simulink model "Different_Functions"  (R2025b)
settings: Solver=FixedStepDiscrete  StartTime=0.0  StopTime=10.0  FixedStep=0.01  RelTol=1e-3
libraries: simulink x1
settings Model: Creator=soura  LastModifiedBy=soura

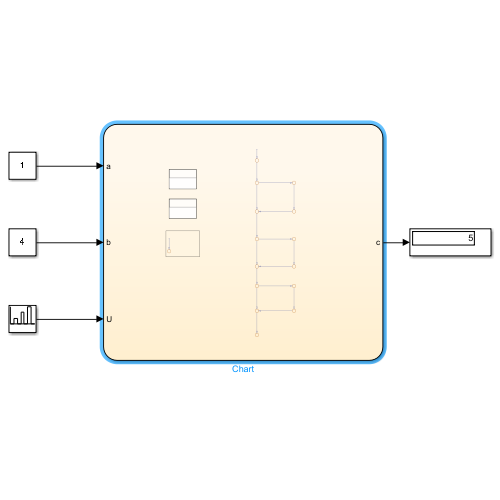
[thumbnail: Simulink's stored preview of the top-level diagram]
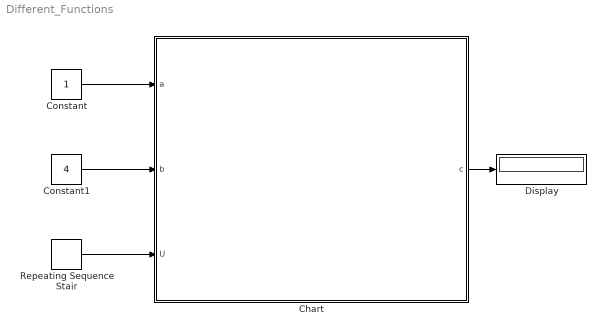
== system Different_Functions ==
  Chart : Stateflow chart  TreatAsAtomicUnit=on
  Constant : Constant  OutDataTypeStr=uint8
  Constant1 : Constant  Value=4  OutDataTypeStr=uint8
  Display : Display
  Repeating Sequence Stair : simulink/Sources/Repeating Sequence Stair  OutValues=[0 1 0 2 0 3 0].'  tsamp=-1  OutMin=[]  OutMax=[]  OutDataTypeStr=double  OutputDataTypeScalingMode=double  OutDataType=fixdt(0,8)  ConRadixGroup=Best Precision: Vector-wise  OutScaling=2^-12
  wires:
  Constant/1 -> Chart/1(a)
  Constant1/1 -> Chart/2(b)
  Repeating Sequence Stair/1 -> Chart/3(U)
  Chart/1(c) -> Display/1

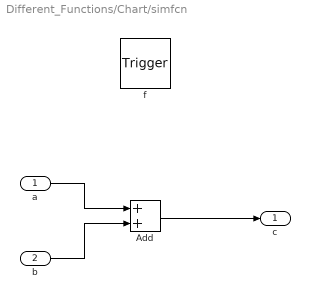
== system Different_Functions/Chart/simfcn ==
  a : Inport  OutDataTypeStr=uint8  PortDimensions=1
  b : Inport  Port=2  OutDataTypeStr=uint8  PortDimensions=1
  f : TriggerPort  TriggerType=function-call  VariantControl=(inherit)
      settings: CopyFcn=Stateflow.SLINSF.SimulinkMan.removeBlockPreDeleteFcn  PreDeleteFcn=Stateflow.SLINSF.SimulinkMan.unsafePredeleteFcn
  Add : Sum
  c : Outport
  wires:
  a/1 -> Add/1
  b/1 -> Add/2
  Add/1 -> c/1

== stateflow chart Different_Functions/Chart ==
  state c = simfcn(a,b) [function]
  state c=add1(a,b) [function]
    (default) -> (junction 14) : {c=a+b;}
  (default) -> (junction 1)
  (junction 1) -> (junction 2) : {c=uint8(0);}
  (junction 2) -> (junction 3) [order 1] : [U==1]
  (junction 2) -> (junction 7) [order 2]
  (junction 3) -> (junction 9) : {c=add(a,b)}
  (junction 9) -> (junction 7)
  (junction 7) -> (junction 21)
  (junction 21) -> (junction 17) [order 1] : [U==2]
  (junction 21) -> (junction 22) [order 2]
  (junction 17) -> (junction 18) : {c = simfcn(a,b)}
  (junction 18) -> (junction 22)
  (junction 22) -> (junction 30)
  (junction 30) -> (junction 19) [order 1] : [U==3]
  (junction 30) -> (junction 47) [order 2]
  (junction 19) -> (junction 20) : {c=add1(a,b)}
  (junction 20) -> (junction 47)
  (junction 47) -> (junction 48)
  data: a function_input; b function_input; c function_output; a function_input uint8 size=1; b function_input uint8 size=1; c function_output; a function_input; b function_input; c function_output; a input uint8; b input uint8; c output; U input
  function c=add(a,b):
    | function c=add(a,b)
    | c=a+b;
    | end
